simulink model "oneWayDiffAdded"  (R2023b)
settings: Solver=VariableStepAuto  StartTime=0.0  StopTime=10.0  RelTol=1e-3
settings Model: Creator=neham  LastModifiedBy=neham

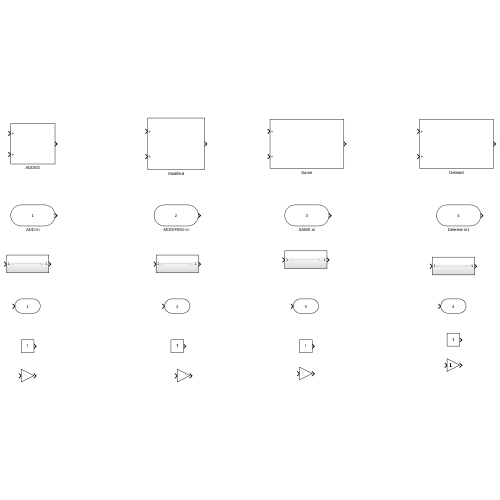
[thumbnail: Simulink's stored preview of the top-level diagram]
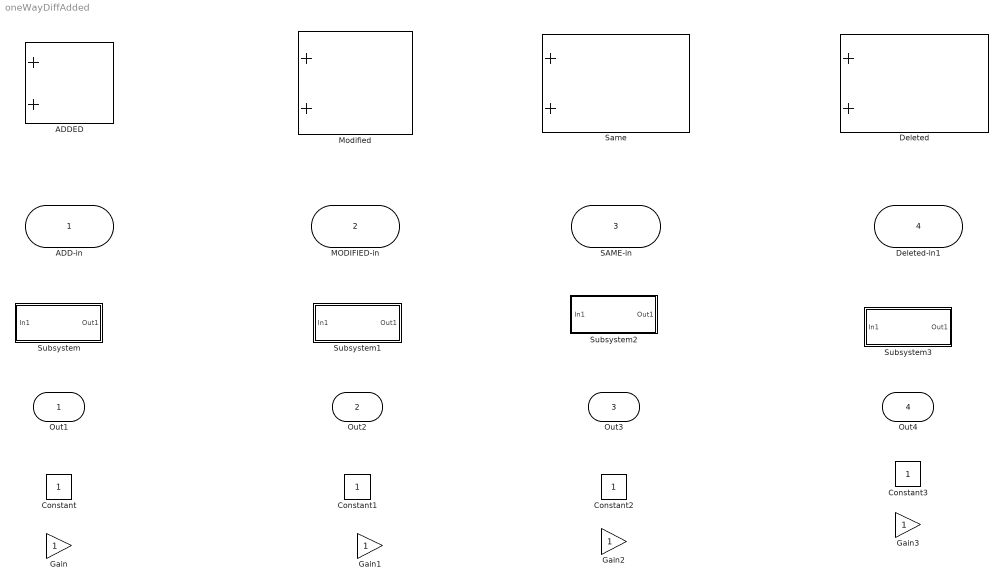
== system oneWayDiffAdded ==
  ADD-in : Inport
  MODIFIED-in : Inport  Port=2
  SAME-in : Inport  Port=3
  Deleted-in1 : Inport  Port=4
  ADDED : Sum
  Constant{,1..3} (4 alike) : Constant
  Deleted : Sum
  Gain{,1..3} (4 alike) : Gain
  Modified : Sum
  Same : Sum
  Subsystem : Subsystem
  Subsystem1 : Subsystem
  Subsystem2 : Subsystem
  Subsystem3 : Subsystem
  Out1 : Outport
  Out2 : Outport  Port=2
  Out3 : Outport  Port=3
  Out4 : Outport  Port=4

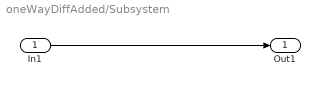
== system oneWayDiffAdded/Subsystem ==
  In1 : Inport
  Out1 : Outport
  wires:
  In1/1 -> Out1/1

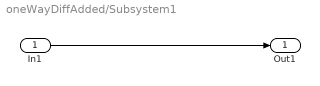
== system oneWayDiffAdded/Subsystem1 ==
  In1 : Inport
  Out1 : Outport
  wires:
  In1/1 -> Out1/1

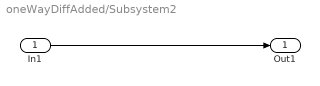
== system oneWayDiffAdded/Subsystem2 ==
  In1 : Inport
  Out1 : Outport
  wires:
  In1/1 -> Out1/1

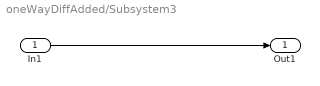
== system oneWayDiffAdded/Subsystem3 ==
  In1 : Inport
  Out1 : Outport
  wires:
  In1/1 -> Out1/1
